simulink model "motorai"  (R2018a)
settings: Solver=FixedStepAuto  StartTime=0.0  StopTime=inf  FixedStep=SAMPLE_TIME  RelTol=1e-3
InitFcn:
  | addpath Functions;
  | addpath Classes;
  | import Parameters.*;
  | 
  | ESTIMATION_SAMPLES = 50;
  | SAMPLE_TIME = 5e-5;
  | DATA_SAMPLING_FREQUENCY  = 500;
  | STEP_VOLTAGE = 5;
  | 
  | motorParameters = Parameters();
  | motorParameters.range('R', [1e-1 1e2]) ...
  |                .range('L', [1e-5 1e-2]) ...
  |                .range('K', [1e-3 1]) ...
  |                .range('f', [1e-7 1e-4]) ...
  |                .range('Jm', [1e-8 1e-4]);
  | 
  | R_ = 65;
  | L_ = 1.41e-3;
  | K_ = 2.55e-2;
  | f_ = 1.11e-7;
  | Jm_ = 7.2e-8;
values from neighbouring files (symbols this model uses):
  Parameters =     [gymmed_test1.mat]
libraries: neural x230, dspbuff3 x2, dspswit3 x1
(part 8 of 11)

== system motorai/Triggered Subsystem/Function Fitting Neural Network1/Layer 2/Delays 1 ==
  "p{2}" : Inport  PortDimensions=166
      mask Display: e = 0.06;c1 = [120 230 180]/255;c2 = ([120 230 180]+0)/(256+128);c3 = ([120 230 180]+128)/(256+128);patch([0 1 1 0],[0 0 1 1],c1);patch([0 1 1 1-e 1-e 0+e],[0 0 1 1-e 0+e 0+e],c2);patch([0 0 1 1-e 0+e 0+e],[0 1 1 1-e 1-e 0+e],c3);plot([0 1 1 0 0],[0 0 1 1 0]);
  mux : Mux  Inputs=1
      mask Display: e = 0.06;c1 = [120 150 230]/255;c2 = ([120 150 230]+0)/383;c3 = ([120 150 230]+128)/383;patch([0 1 1 0],[0 0 1 1],c1);patch([0 1 1 1-e 1-e 0+e],[0 0 1 1-e 0+e 0+e],c2);patch([0 0 1 1-e 0+e 0+e],[0 1 1 1-e 1-e 0+e],c3);plot([0 1 1 0 0],[0 0 1 1 0]);disp('Mux')
  "pd{2,1}" : Outport
      mask Display: e = 0.06;c1 = [120 230 180]/255;c2 = ([120 230 180]+0)/(256+128);c3 = ([120 230 180]+128)/(256+128);patch([0 1 1 0],[0 0 1 1],c1);patch([0 1 1 1-e 1-e 0+e],[0 0 1 1-e 0+e 0+e],c2);patch([0 0 1 1-e 0+e 0+e],[0 1 1 1-e 1-e 0+e],c3);plot([0 1 1 0 0],[0 0 1 1 0]);
  wires:
  "p{2}"/1 -> mux/1
  mux/1 -> "pd{2,1}"/1
